simulink model "displayTest"  (R2022b)
settings: Solver=FixedStepDiscrete  StartTime=0.0  StopTime=10.0  FixedStep=0.01  RelTol=1e-3  EnableMultiTasking=on
PreLoadFcn:
  | try, model_open; catch, disp('Error occurred while executing model pre-load callback: model_open.m'); disp('Please assure that the MATLAB working directory is set to the model directory before opening.'); end
InitFcn:
  | try, model_open; catch, end
model workspace (MAT data in the model file):
  IOScreen_Label_XCoord = 1
  IOScreen_Row1_YCoord = 1
  IOScreen_Row2_YCoord = 12
  IOScreen_Value_XCoord = 110
  MainScreen_Row1_YCoord = 7
  MainScreen_Row2_YCoord = 23
  MainScreen_Symbols_XCoord = 1
  MainScreen_Units_XCoord = 69
  MainScreen_Value_XCoord = 64
undefined symbols (not defined in the file or in its folder): curr_screen, DISP, gesture, raptor_get_buildNum, raptor_get_safe_string, raptor_hwexp, raptor_xcp_function, Screens, VC500
libraries: Raptor_display_lib x93, Raptor_lib x40, Raptor_Datalogging_lib x10, simulink_extras x3, simulink x2
(part 3 of 3)

== system displayTest/Foreground/Display/Screens/Navigation/Go Right/IO ==
  Action Port : ActionPort  ActionPortLabel=case [ 2 ]:
  display_goto_screen : Raptor_display_lib/Screen Functions/display_goto_screen  screenPort=off  ScreenName='MainScreen'
      settings: SourceProductName=Raptor Display Library

== system displayTest/Foreground/Display/Screens/Navigation/Go Right/Main ==
  Action Port : ActionPort  ActionPortLabel=case [ 1 ]:
  display_goto_screen : Raptor_display_lib/Screen Functions/display_goto_screen  screenPort=off  ScreenName='AboutScreen'
      settings: SourceProductName=Raptor Display Library

== system displayTest/Foreground/Display/Data Logging/Write to Log/Open Existing File/File Seek/File Open Failure ==
  file_in : Inport
  Enable : EnablePort
  Constant : Constant  Value=false  OutDataTypeStr=Inherit: Inherit via back propagation
  file_out : Outport  VectorParamsAs1DForOutWhenUnconnected=off
  Success : Outport  Port=2  VectorParamsAs1DForOutWhenUnconnected=off
  wires:
  Constant/1 -> Success/1
  file_in/1 -> file_out/1

== system displayTest/Foreground/Display/Data Logging/Write to Log/Open Existing File/File Seek/File Open Success ==
  file_in : Inport
  Enable : EnablePort
  Constant : Constant  Value=0  OutDataTypeStr=Inherit: Inherit via back propagation
  raptor_fileIO_seek1 : Raptor_Datalogging_lib/raptor_fileIO_seek  resourceValues=USB|(None)  resource=USB  seekTypeValues=File Start|Current Location|File End  seekType=3
      settings: SourceProductName=Raptor Data Logging
  file_out : Outport  VectorParamsAs1DForOutWhenUnconnected=off
  Out2 : Outport  Port=2  VectorParamsAs1DForOutWhenUnconnected=off
  wires:
  raptor_fileIO_seek1/1 -> file_out/1
  raptor_fileIO_seek1/2 -> Out2/1
  file_in/1 -> raptor_fileIO_seek1/1
  Constant/1 -> raptor_fileIO_seek1/2

== system displayTest/Foreground/Display/Screens/DataLogScreen_Update/Element/Toggle Switch1/Triggered Subsystem ==
  Trigger : TriggerPort  VariantControl=Variant
  Constant2 : Constant
  D Latch : simulink_extras/Flip Flops/D Latch
  Unit Delay : UnitDelay  InitialCondition=InitialCondition  SampleTime=-1  HasFrameUpgradeWarning=on
  Out1 : Outport  VectorParamsAs1DForOutWhenUnconnected=off
  wires:
  D Latch/2 -> Unit Delay/1
  Unit Delay/1 -> D Latch/1
  D Latch/1 -> Out1/1
  Constant2/1 -> D Latch/2

== system displayTest/Foreground/Display/Screens/IOScreen_Update/IOElement1/Toggle Switch1/Triggered Subsystem ==
  Trigger : TriggerPort  VariantControl=Variant
  Constant2 : Constant
  D Latch : simulink_extras/Flip Flops/D Latch
  Unit Delay : UnitDelay  InitialCondition=InitialCondition  SampleTime=-1  HasFrameUpgradeWarning=on
  Out1 : Outport  VectorParamsAs1DForOutWhenUnconnected=off
  wires:
  D Latch/2 -> Unit Delay/1
  Unit Delay/1 -> D Latch/1
  D Latch/1 -> Out1/1
  Constant2/1 -> D Latch/2

== system displayTest/Foreground/Display/Screens/IOScreen_Update/IOElement1/Toggle Switch2/Triggered Subsystem ==
  Trigger : TriggerPort  VariantControl=Variant
  Constant2 : Constant
  D Latch : simulink_extras/Flip Flops/D Latch
  Unit Delay : UnitDelay  InitialCondition=InitialCondition  SampleTime=-1  HasFrameUpgradeWarning=on
  Out1 : Outport  VectorParamsAs1DForOutWhenUnconnected=off
  wires:
  Constant2/1 -> D Latch/2
  D Latch/1 -> Out1/1
  Unit Delay/1 -> D Latch/1
  D Latch/2 -> Unit Delay/1
